simulink model "hw3_1c_ActivationDependentCE"  (R2013a)
settings: Solver=ode45  StartTime=0.0  StopTime=runtime  MaxStep=0.01  RelTol=1e-3
InitFcn:
  | % f-L relationship
  | lopt = 0.08;
  | w = 0.56*lopt;
  | 
  | % f-v relationship
  | K = 5;
  | N = 1.5;
  | vmax = -12*lopt; % m/s, typically expressed as a negative number when talking abotu contraction
  | 
  | % max isometric force
  | Fmax = 6000; % N
  | 
  | % reference strain
  | e_ref = w*2;
  | 
  | runtime = 10;
libraries: simulink x3
settings Model: Creator=benshih  LastModifiedBy=benshih

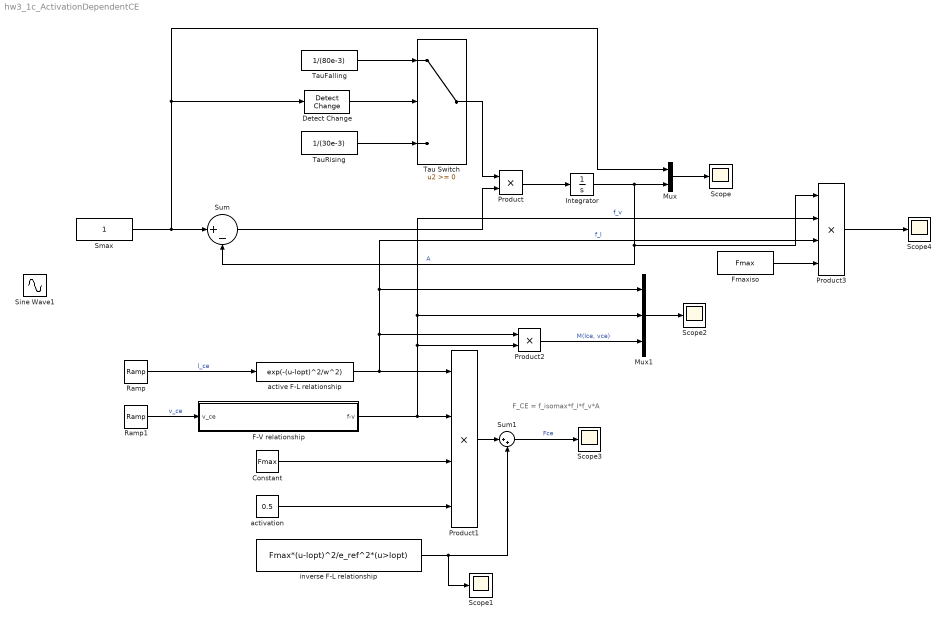
== system hw3_1c_ActivationDependentCE ==
  note: F_CE = f_isomax*f_l*f_v*A
  Constant : Constant  Value=Fmax
  Detect Change : simulink/Logic and Bit Operations/Detect Change  vinit=0  InputProcessing=Inherited  OutDataTypeStr=uint8
  F-V relationship : Subsystem
  Fmaxiso : Constant  Value=Fmax
  Integrator : Integrator
  Mux : Mux  Inputs=2
  Mux1 : Mux  Inputs=3
  Product : Product
  Product1 : Product  Inputs=4
  Product2 : Product
  Product3 : Product  Inputs=4
  Ramp : simulink/Sources/Ramp  slope=2*lopt/runtime  start=0  X0=0
  Ramp1 : simulink/Sources/Ramp  slope=-vmax*2/runtime  start=0  X0=vmax
  Scope{,1..4} (5 alike) : Scope
      Scope1 settings: SaveName=ScopeData5
      Scope2 settings: SaveName=ScopeData4
      Scope3 settings: SaveName=ScopeData2
      Scope4 settings: SaveName=ScopeData6
  Sine Wave1 : Sin  Amplitude=1/2  Bias=1/2  Frequency=2*pi*5  SampleTime=0
  Smax : Constant
  Sum : Sum  Inputs=|+-
  Sum1 : Sum  Inputs=|++
  Tau Switch : Switch
  TauFalling : Constant  Value=1/(80e-3)
  TauRising : Constant  Value=1/(30e-3)
  activation : Constant  Value=0.5
  active F-L relationship : Fcn  Expr=exp(-(u-lopt)^2/w^2)
  inverse F-L relationship : Fcn  Expr=Fmax*(u-lopt)^2/e_ref^2*(u>lopt)
  wires:
  Smax/1 -> Mux/1, Detect Change/1, Sum/1
  Integrator/1 -> Mux/2, Sum/2, Product3/1  "A"
  TauFalling/1 -> Tau Switch/1
  TauRising/1 -> Tau Switch/3
  Detect Change/1 -> Tau Switch/2
  Sum/1 -> Product/2
  Tau Switch/1 -> Product/1
  Product/1 -> Integrator/1
  Mux/1 -> Scope/1
  Ramp/1 -> active F-L relationship/1  "l_ce"
  active F-L relationship/1 -> Product3/3, Mux1/1, Product2/1, Product1/1  "f_l"
  Ramp1/1 -> F-V relationship/1(v_ce)  "v_ce"
  F-V relationship/1(f-v) -> Product3/2, Mux1/2, Product2/2, Product1/2  "f_v"
  Constant/1 -> Product1/3
  activation/1 -> Product1/4
  Product1/1 -> Sum1/1
  inverse F-L relationship/1 -> Scope1/1, Sum1/2
  Sum1/1 -> Scope3/1  "Fce"
  Product2/1 -> Mux1/3  "M(lce, vce)"
  Mux1/1 -> Scope2/1
  Fmaxiso/1 -> Product3/4
  Product3/1 -> Scope4/1

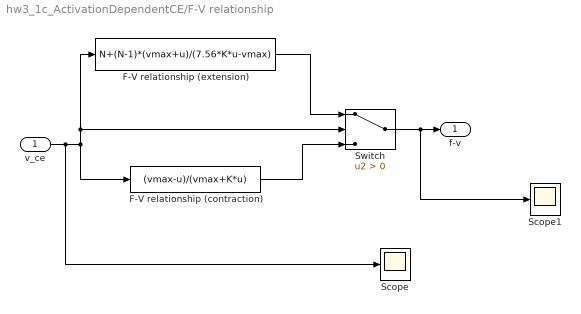
== system hw3_1c_ActivationDependentCE/F-V relationship ==
  v_ce : Inport
  F-V relationship (contraction) : Fcn  Expr=(vmax-u)/(vmax+K*u)
  F-V relationship (extension) : Fcn  Expr=N+(N-1)*(vmax+u)/(7.56*K*u-vmax)
  Scope : Scope
  Scope1 : Scope
      settings: SaveName=ScopeData3
  Switch : Switch  Criteria=u2 > Threshold
  f-v : Outport
  wires:
  v_ce/1 -> Scope/1, F-V relationship (extension)/1, Switch/2, F-V relationship (contraction)/1
  Switch/1 -> Scope1/1, f-v/1
  F-V relationship (extension)/1 -> Switch/1
  F-V relationship (contraction)/1 -> Switch/3
